simulink subsystem "Circuit_5State_Noise_fnc_StateNoise"  (R2022a)
settings: Solver=VariableStepAuto  StartTime=0.0  StopTime=10.0  RelTol=1e-3
values from neighbouring files (symbols this model uses):
  C_m = C_des(1,:)    [RunNoisyPlant.m]
  K_plant = LC_param.K    [RunNoisyPlant.m]
  M_cross = LC_param.M_cross    [RunNoisyPlant.m]    (also in getLCParam.m = V*S_cross*U')
  SV_IC = SIM.x_0    [RunNoisyPlant.m]
  tc = 1e-7    (= 1e-07)    [RunNoisyPlant.m]
  Ts = 1e-6    (= 1e-06)    [RunNoisyPlant.m]
  U_NV_NT = LC_param.U_NV_NT    [RunNoisyPlant.m]    (also in getLCParam.m = U_null*V_null')
undefined symbols (not defined in the file or in its folder): FLAG, N, P, SIM
libraries: simulink x2
settings Model: Creator=tyevans  LastModifiedBy=tyevans

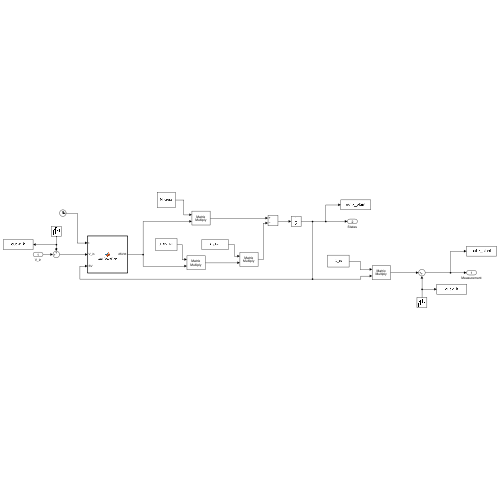
[thumbnail: Simulink's stored preview of the top-level diagram]
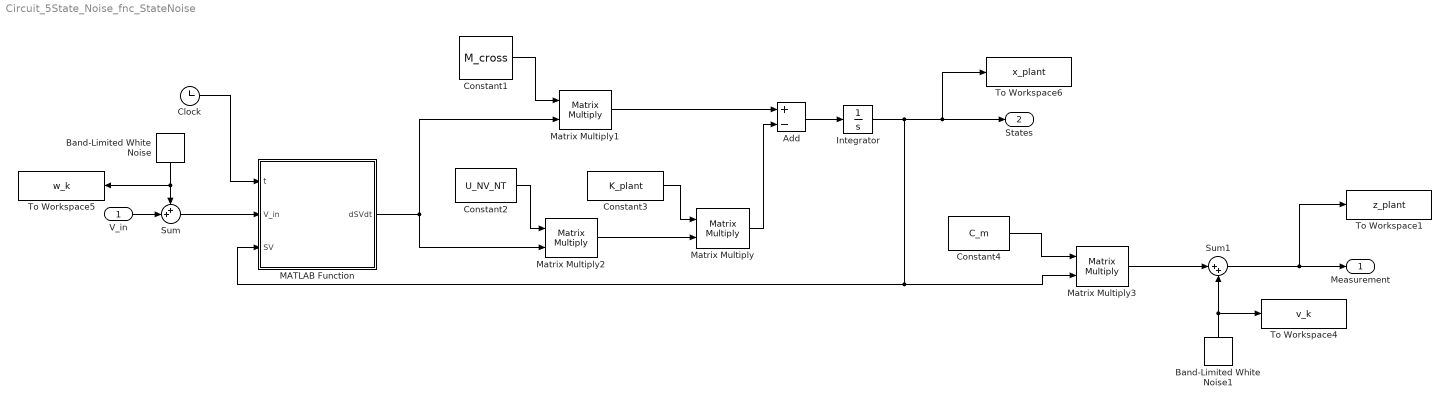
== system Circuit_5State_Noise_fnc_StateNoise ==
  V_in : Inport
  Add : Sum  Inputs=+-
  Band-Limited White Noise : simulink/Sources/Band-Limited White Noise  Cov=pow_Q  Ts=tc  seed=[1]  VectorParams1D=off
  Band-Limited White Noise1 : simulink/Sources/Band-Limited White Noise  Cov=pow_R  Ts=tc  seed=[23341]  VectorParams1D=off
  Clock : Clock
  Constant1 : Constant  Value=M_cross  VectorParams1D=off
  Constant2 : Constant  Value=U_NV_NT  VectorParams1D=off
  Constant3 : Constant  Value=K_plant  VectorParams1D=off
  Constant4 : Constant  Value=C_m  VectorParams1D=off
  Integrator : Integrator  InitialCondition=SV_IC
  MATLAB Function : MATLAB Function  TreatAsAtomicUnit=on
  Matrix Multiply{,1..3} (4 alike) : Product  Multiplication=Matrix(*)
  Sum : Sum  Inputs=++|
  Sum1 : Sum  Inputs=|++
  To Workspace1 : ToWorkspace  VariableName=z_plant  SaveFormat=Structure With Time  SampleTime=Ts
  To Workspace4 : ToWorkspace  VariableName=v_k  SaveFormat=Structure With Time  SampleTime=-1
  To Workspace5 : ToWorkspace  VariableName=w_k  SaveFormat=Structure With Time  SampleTime=-1
      settings: Save2DSignal=2-D array (concatenate along first dimension)
  To Workspace6 : ToWorkspace  VariableName=x_plant  SaveFormat=Structure With Time  SampleTime=Ts
  Measurement : Outport
  States : Outport  Port=2
  wires:
  V_in/1 -> Sum/2
  Band-Limited White Noise/1 -> To Workspace5/1, Sum/1
  Sum1/1 -> Measurement/1, To Workspace1/1
  Band-Limited White Noise1/1 -> To Workspace4/1, Sum1/2
  Clock/1 -> MATLAB Function/1(t)
  Sum/1 -> MATLAB Function/2(V_in)
  Matrix Multiply3/1 -> Sum1/1
  Constant1/1 -> Matrix Multiply1/1
  Constant2/1 -> Matrix Multiply2/1
  Matrix Multiply1/1 -> Add/1
  Add/1 -> Integrator/1
  Constant4/1 -> Matrix Multiply3/1
  Matrix Multiply/1 -> Add/2
  Constant3/1 -> Matrix Multiply/1
  MATLAB Function/1(dSVdt) -> Matrix Multiply1/2, Matrix Multiply2/2
  Integrator/1 -> To Workspace6/1, States/1, MATLAB Function/3(SV), Matrix Multiply3/2
  Matrix Multiply2/1 -> Matrix Multiply/2

== matlab function Circuit_5State_Noise_fnc_StateNoise/MATLAB Function ==
  data: t input; dSVdt output; V_in input; SV input; SIM parameter; N parameter; P parameter; FLAG parameter
function dSVdt = CallGovnEqn(t,V_in, SV,SIM, N, P, FLAG)
% Initialize Output
dSVdt = zeros(N.states,1);

% Call Governing Equations
[dSVdt] = DAECircGovnEqn(t,SV,SIM,N,P,FLAG,V_in);
end
